simulink model "Faultframework"  (R2014a)
settings: Solver=FixedStepDiscrete  StartTime=0.0  StopTime=SimLength  FixedStep=SampleTime  RelTol=1e-3
PreLoadFcn:
  | set_global_callback;
settings Model: Creator=georg  LastModifiedBy=georg

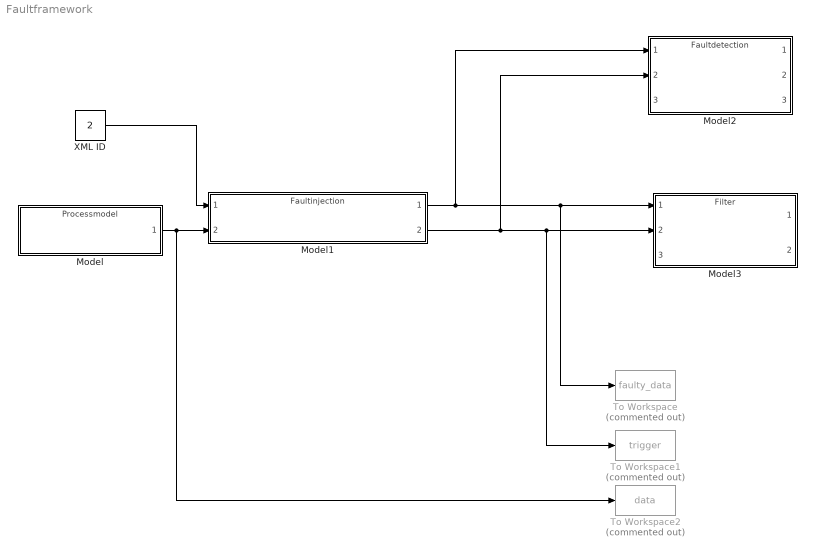
== system Faultframework ==
  Model : ModelReference  ModelNameDialog=Processmodel.slx  SimulationMode=Normal  ModelReferenceVersion=1.12  CopyOfModelName=Processmodel.slx  DefaultDataLogging=on
  Model1 : ModelReference  ModelNameDialog=Faultinjection.slx  SimulationMode=Normal  ModelReferenceVersion=1.10  CopyOfModelName=Faultinjection.slx  DefaultDataLogging=on
  Model2 : ModelReference  ModelNameDialog=Faultdetection.slx  SimulationMode=Normal  ModelReferenceVersion=1.44  CopyOfModelName=Faultdetection.slx  DefaultDataLogging=on
  Model3 : ModelReference  ModelNameDialog=Filter  SimulationMode=Normal  ModelReferenceVersion=1.24  CopyOfModelName=Filter  DefaultDataLogging=on
  To Workspace : ToWorkspace  Commented=on  VariableName=faulty_data  SaveFormat=Timeseries  SampleTime=-1
  To Workspace1 : ToWorkspace  Commented=on  VariableName=trigger  SaveFormat=Timeseries  SampleTime=-1
  To Workspace2 : ToWorkspace  Commented=on  VariableName=data  SaveFormat=Timeseries  SampleTime=-1
  XML ID : Constant  Value=2  OutDataTypeStr=single
  wires:
  Model/1 -> To Workspace2/1, Model1/2
  Model1/1 -> Model2/1, To Workspace/1, Model3/1
  XML ID/1 -> Model1/1
  Model1/2 -> Model2/2, To Workspace1/1, Model3/2
